simulink model "Series"  (R2020a)
settings: Solver=VariableStepAuto  StartTime=0.0  StopTime=6948  RelTol=1e-3
values from neighbouring files (symbols this model uses):
  diff_gear = 4.51    [Series_script.m]
  gear_down = []    [Series_script.m]
  gear_eff = 0.98    [Series_script.m]
  gear_idling_loss = 0    [Series_script.m]
  gear_ratio = [1]    [Series_script.m]
  gear_up = []    [Series_script.m]
  Gears = 1    [Series_script.m]
  max_battery = 0.6*150*1000    (= 90000)    [Series_script.m]
  max_CE_power = 48    [Series_script.m]
  max_EG_power = 35    [Series_script.m]
  max_EM_power = 150    [Series_script.m]
  max_SOC = 0.60    (= 0.6)    [Series_script.m]
  min_SOC = 0.30    (= 0.3)    [Series_script.m]
  Series_add_Mass = 250    [Series_script.m]
  T_CE_max = p_me_max.*V_d/(2*pi*2)    [Eng_plot.m]
  T_EG_max = max_EG_power *1000 / max_EG_power_old * T_EG_max    [Gen_plot.m]
  T_EM_max = max_EM_power *1000 / max_EM_power_old * T_EM_max    [motor_plot.m]
  V_Mass = 1920    [Series_script.m]
  V_wheel_dia = 0.739    [Series_script.m]
undefined symbols (not defined in the file or in its folder): automatic_gearbox, eta_EG_map, eta_EM_map, H_u, P_aux, P_CE_cutoff, P_CE_idle, r, T_CE_cutoff, theta_CE, theta_EM, V_CE_map, w_CE_idle, w_CE_max, w_CE_upper, w_EG_row, w_EG_upper, w_EM_row, w_EM_upper
libraries: qss_tb_library x6, simulink x1
settings Model: Creator=Rahul Pai  LastModifiedBy=Rahul Pai

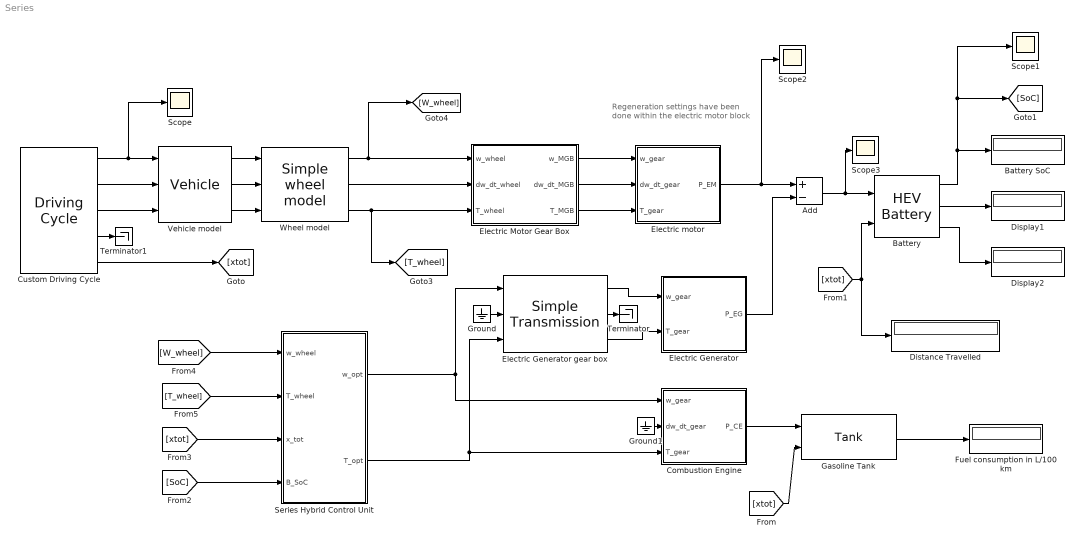
== system Series ==
  note: Regeneration settings have been
      | done within the electric motor block
  Add : Sum  Inputs=+-
  Battery : qss_tb_library/Energy Buffer/HEV Battery  Tag=battery  cell_series=N_series  cell_parallel=N_parallel  Q_BT_IC_rel=Init_SoC
  Battery SoC : Display
  Combustion Engine : Subsystem  Tag=combustion engine  AncestorBlock=qss_tb_library/Energy Converter/CE Assignment  mask(Combustion Engine (based on consumption map)){engine_type=Gasoline, P_ice=max_CE_power, ENABLE_FUEL_CUTOFF=on}
      mask prompts: engine_type "Engine type"; P_ice "Power [kW]"; ENABLE_FUEL_CUTOFF "Enable fuel cutoff"
      mask help:
      | This block simulates the behaviour of a combustion engine. The block is based on consumption maps for medium sized passenger cars.
      |
      | NA Gasoline:
      | max power @ 5000 rpm
      | max torque @ 3000 rpm
      |
      | Small Diesel:
      | max power @ 4500 rpm
      | max torque @ 2000 rpm
      |
      | Large Diesel:
      | max power @ 1500 rpm
      | max torque @ 1500 rpm
      |
      |
      | Input:
      | =====
      | 	w_gear	Speed of the fly wheel [rad/s]
      | 	dw_dt_gear	Acceleration of the fly wheel [rad/s^2]
      | 	T_gear	Torque on the fly wheel [Nm]
      |
      | Output:
      | ======
      | 	P_CE	Fuel power consumed by the combustion engine [W]
      mask init:
      | init_AssCE_map;
      mask TypeOptions engine_type: Gasoline | Small Diesel | Large Diesel
  Custom Driving Cycle : qss_tb_library/Driving Cycle/Driving Cycle  Tag=cycle  cyclename1=Assignment_2_cycle  stepsize=1  autostop=on
  Display1 : Display
  Display2 : Display
  Distance Travelled : Display
      settings: Format=decimal (Stored Integer)
  Electric Generator : Subsystem  AncestorBlock=qss_tb_library/Energy Converter/EG Assignment  mask(Electric Generator){P_eg=max_EG_power}
      mask prompts: P_eg "Maximum mechanical power [kW]"
      mask help:
      | This block simulates the behaviour of an electric generator. The block is based on an efficiency map.
      |
      | Input:
      | =====
      | 	w_gear	Speed of the generator [rad/s]
      | 	T_gear	Torque of the generator [Nm]
      |
      | Output:
      | ======
      | 	P_EG	Electric power of the generator [W]
      |
      | Generator map:
      | ======
      | The generator map file must contain the following variables:
      | eta_EG_map		% Efficiency map                    [-]
      | w_EG_row                        % Generator speed range             [rad/s]
      | T_EG_col		% Generator torque range            [Nm]
      | w_EG_max		% Maximum generator speed           [rad/s]
      | T_EG_max		% Maximum generator torque          [Nm]
      |
      | ======
      mask init:
      | init_EG_ass;
  Electric Generator gear box : qss_tb_library/Gear System/Simple Transmission  Tag=simple transmission  gear_ratio=EM_gear_ratio  e_GT=EM_gear_eta  P_GT0=EM_idling_loss  w_wheel_min=1
  Electric Motor Gear Box : Subsystem  Tag=transmission  AncestorBlock=qss_tb_library/Gear System/Automatic Gear Box  mask(Automatic Gear Box){nog=Gears, i=gear_ratio, i_diff=diff_gear, gearon=gear_up, gearoff=gear_down, d=V_wheel_dia, e_GT=gear_eff, P_GT0=gear_idling_loss, w_wheel_min=1}
      mask prompts: nog "Number of gears"; i "Gear ratio vector"; i_diff "Differential gear [-]"; gearon "Switching points for upshift [km/h]"; gearoff "Switching points for downshift [km/h]"; d "Wheel diameter"; e_GT "Efficiency [-]"; P_GT0 "Idling losses (friction) [W]"; w_wheel_min "Minimum wheel speed beyond which losses are generated [rad/s]"
      mask help:
      | This block simulates a automatic gear box, can handle up to 16 gears.
      |
      | Input:
      | =====
      | 	w_wheel	Speed of the wheel [rad/s]
      | 	dw_dt_wheel	Acceleration of the wheel [rad/s^2],
      | 	T_wheel	Torque on the wheel [Nm]
      | 	i	Gear number [-]
      |
      | Output:
      | ======
      | 	w_MGB	Speed of the fly wheel [rad/s]
      | 	dw_dt_MGB	Acceleration of the fly wheel [rad/s^2]
      | 	T_MGB	Torque on the fly wheel [Nm]
      |
      | Number of gears:
      | ======
      | Specify the number of forward gears
      |
      | Shifting points for upshift:
      | ======
      | Vector specifying the velocity for shifting
      | [first_to_second_gear    second_to_third_gear    ....]
      | The number of elements in the vector should be Number of gears - 1.
      |
      | Shifting points for udownshift:
      | ======
      | Simular to upshift
      | [second_to_first_gear    third_to_second_gear    ....]
      mask init:
      | init_AGB;
  Electric motor : Subsystem  AncestorBlock=qss_tb_library/Energy Converter/EM Assignment  mask(Electric Motor){P_em=max_EM_power}
      mask prompts: P_em "Power [kW]"
      mask help:
      | This block simulates the behaviour of an electric motor. The block is based on an efficiency map. The map is located in the Data/EnergyConvertter/ElectricMotor directory.
      |
      | Maximum speed och the electric motor is 6000 rpm
      | Field weakening region starts at 1500 rpm
      | Maximum mechanical power is at 2150 rpm
      | The maximum torque is 5.98 Nm/kW multiplied with the power you select.
      |
      | Input:
      | =====
      | 	w_gear	Speed of the motor [rad/s]
      | 	dw_dt_gear	Acceleration of the motor [rad/s^2]
      | 	T_gear	Torque of the motor [Nm]
      |
      | Output:
      | ======
      | 	P_EM	Electric Power consumed by the  motor [W]
      mask init:
      | init_EM_ass;
  Fuel consumption in L/100 km : Display
  Gasoline Tank : qss_tb_library/Energy Source/Tank  Tag=tank  fuel=Gasoline  flag_cold_start=on
  Ground : Ground
  Ground1 : Ground
  Scope{,1..3} (4 alike) : Scope
  Series Hybrid Control Unit : Subsystem  Tag=control unit  AncestorBlock=|  mask(Control Unit){}
      | qss_tb_library/Controller/Control Unit
      | (empty template)
      mask help:
      | This block gives the user the opportunity to design his/her own control unit.
      |
      | The user can define the inputs and outputs  by himself/herself.
  Terminator : Terminator
  Terminator1 : Terminator
  Vehicle model : qss_tb_library/Vehicle/Vehicle  Tag=vehicle  m_f=V_Mass+Series_add_Mass  A_f=V_area  cw=V_d  mu=V_RRC  k_inertia=V_Rotating
  Wheel model : qss_tb_library/Vehicle/Simple wheel model  Tag=simple transmission  d_wheel=V_wheel_dia
  wires:
  Custom Driving Cycle/1 -> Scope/1, Vehicle model/1
  Custom Driving Cycle/2 -> Vehicle model/2
  Custom Driving Cycle/3 -> Vehicle model/3
  Vehicle model/1 -> Wheel model/1
  Vehicle model/2 -> Wheel model/2
  Vehicle model/3 -> Wheel model/3
  Wheel model/1 -> [W_wheel], Electric Motor Gear Box/1(w_wheel)
  Wheel model/2 -> Electric Motor Gear Box/2(dw_dt_wheel)
  Electric Motor Gear Box/1(w_MGB) -> Electric motor/1(w_gear)
  Electric Motor Gear Box/2(dw_dt_MGB) -> Electric motor/2(dw_dt_gear)
  Electric Motor Gear Box/3(T_MGB) -> Electric motor/3(T_gear)
  Electric motor/1(P_EM) -> Scope2/1, Add/1
  Battery/1 -> Scope1/1, [SoC], Battery SoC/1
  Battery/2 -> Display1/1
  Battery/3 -> Display2/1
  Gasoline Tank/1 -> Fuel consumption in L/100 km/1
  Combustion Engine/1(P_CE) -> Gasoline Tank/1
  Electric Generator gear box/1 -> Electric Generator/1(w_gear)
  Electric Generator gear box/3 -> Electric Generator/2(T_gear)
  Electric Generator gear box/2 -> Terminator/1
  Ground/1 -> Electric Generator gear box/2
  Ground1/1 -> Combustion Engine/2(dw_dt_gear)
  Custom Driving Cycle/5 -> [xtot]
  [xtot] -> Gasoline Tank/2
  [xtot] -> Battery/2, Distance Travelled/1
  Electric Generator/1(P_EG) -> Add/2
  Add/1 -> Scope3/1, Battery/1
  Series Hybrid Control Unit/1(w_opt) -> Combustion Engine/1(w_gear), Electric Generator gear box/1
  Series Hybrid Control Unit/2(T_opt) -> Electric Generator gear box/3, Combustion Engine/3(T_gear)
  [SoC] -> Series Hybrid Control Unit/4(B_SoC)
  [xtot] -> Series Hybrid Control Unit/3(x_tot)
  Wheel model/3 -> [T_wheel], Electric Motor Gear Box/3(T_wheel)
  Custom Driving Cycle/4 -> Terminator1/1
  [T_wheel] -> Series Hybrid Control Unit/2(T_wheel)
  [W_wheel] -> Series Hybrid Control Unit/1(w_wheel)

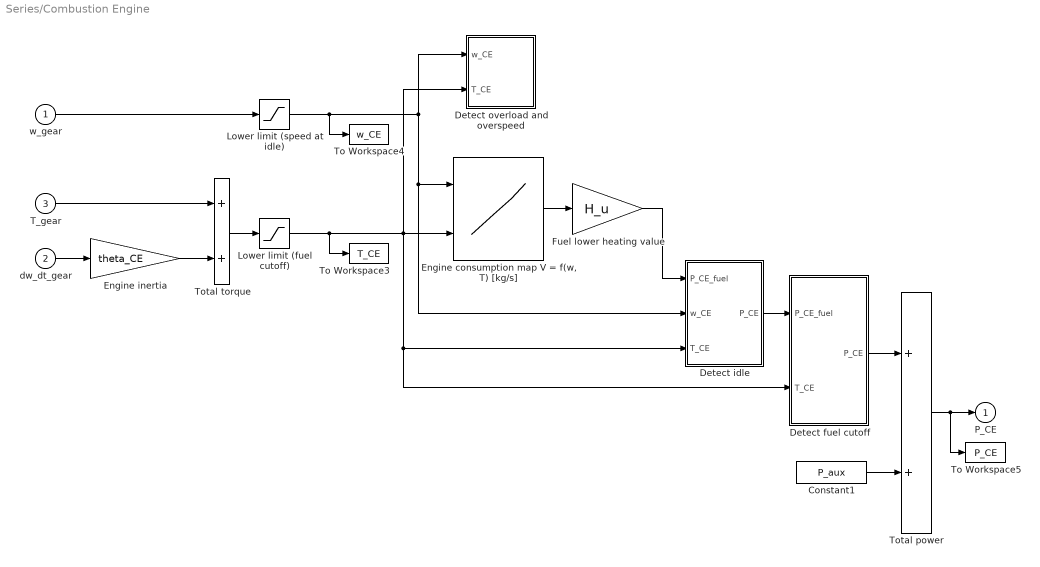
== system Series/Combustion Engine ==
  w_gear : Inport
  dw_dt_gear : Inport  Port=2
  T_gear : Inport  Port=3
  Constant1 : Constant  Value=P_aux
  Detect fuel cutoff : Subsystem
  Detect idle : Subsystem
  Detect overload and overspeed : Subsystem
  "Engine consumption map V = f(w, T) [kg/s]" : Lookup2D  RowIndex=w_CE_row  ColumnIndex=T_CE_col  Table=V_CE_map
  Engine inertia : Gain  Gain=theta_CE  SaturateOnIntegerOverflow=on  OutDataTypeStr=Inherit: Same as input  ParamDataTypeStr=Inherit: Same as input
  Fuel lower heating value : Gain  Gain=H_u  SaturateOnIntegerOverflow=on  OutDataTypeStr=Inherit: Same as input  ParamDataTypeStr=Inherit: Same as input
  Lower limit (fuel cutoff) : Saturate  UpperLimit=inf  LowerLimit=T_CE_cutoff
  Lower limit (speed at idle) : Saturate  UpperLimit=inf  LowerLimit=w_CE_idle
  To Workspace3 : ToWorkspace  VariableName=T_CE  SampleTime=-1
  To Workspace4 : ToWorkspace  VariableName=w_CE  SampleTime=-1
  To Workspace5 : ToWorkspace  VariableName=P_CE  SampleTime=-1
  Total power : Sum  InputSameDT=on  SaturateOnIntegerOverflow=on  OutDataTypeStr=Inherit: Same as first input
  Total torque : Sum  InputSameDT=on  SaturateOnIntegerOverflow=on  OutDataTypeStr=Inherit: Same as first input
  P_CE : Outport  InitialOutput=0
  wires:
  T_gear/1 -> Total torque/1
  dw_dt_gear/1 -> Engine inertia/1
  Total torque/1 -> Lower limit (fuel cutoff)/1
  Engine inertia/1 -> Total torque/2
  Lower limit (speed at idle)/1 -> Detect overload and overspeed/1(w_CE), Detect idle/2(w_CE), "Engine consumption map V = f(w, T) [kg/s]"/1, To Workspace4/1
  w_gear/1 -> Lower limit (speed at idle)/1
  Fuel lower heating value/1 -> Detect idle/1(P_CE_fuel)
  Detect idle/1(P_CE) -> Detect fuel cutoff/1(P_CE_fuel)
  "Engine consumption map V = f(w, T) [kg/s]"/1 -> Fuel lower heating value/1
  Detect fuel cutoff/1(P_CE) -> Total power/1
  Total power/1 -> P_CE/1, To Workspace5/1
  Constant1/1 -> Total power/2
  Lower limit (fuel cutoff)/1 -> Detect overload and overspeed/2(T_CE), "Engine consumption map V = f(w, T) [kg/s]"/2, Detect idle/3(T_CE), Detect fuel cutoff/2(T_CE), To Workspace3/1

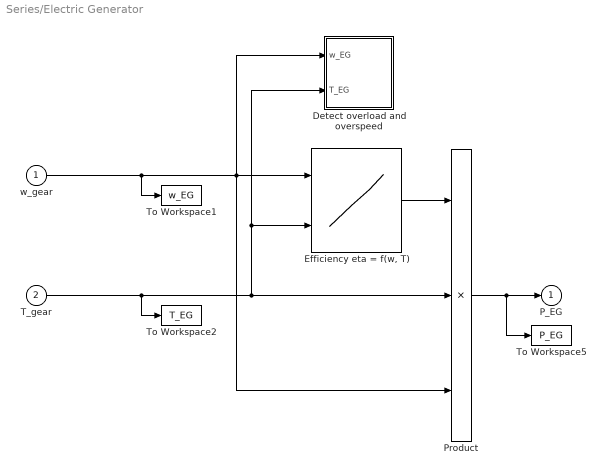
== system Series/Electric Generator ==
  w_gear : Inport
  T_gear : Inport  Port=2
  Detect overload and overspeed : Subsystem
  "Efficiency eta = f(w, T)" : Lookup2D  RowIndex=w_EG_row  ColumnIndex=T_EG_col  Table=eta_EG_map
  Product : Product  Inputs=3  InputSameDT=on  RndMeth=Zero  SaturateOnIntegerOverflow=on  OutDataTypeStr=Inherit: Same as first input
  To Workspace1 : ToWorkspace  VariableName=w_EG  SampleTime=-1
  To Workspace2 : ToWorkspace  VariableName=T_EG  SampleTime=-1
  To Workspace5 : ToWorkspace  VariableName=P_EG  SampleTime=-1
  P_EG : Outport  InitialOutput=0
  wires:
  w_gear/1 -> To Workspace1/1, Detect overload and overspeed/1(w_EG), "Efficiency eta = f(w, T)"/1, Product/3
  Product/1 -> To Workspace5/1, P_EG/1
  "Efficiency eta = f(w, T)"/1 -> Product/1
  T_gear/1 -> To Workspace2/1, Detect overload and overspeed/2(T_EG), "Efficiency eta = f(w, T)"/2, Product/2

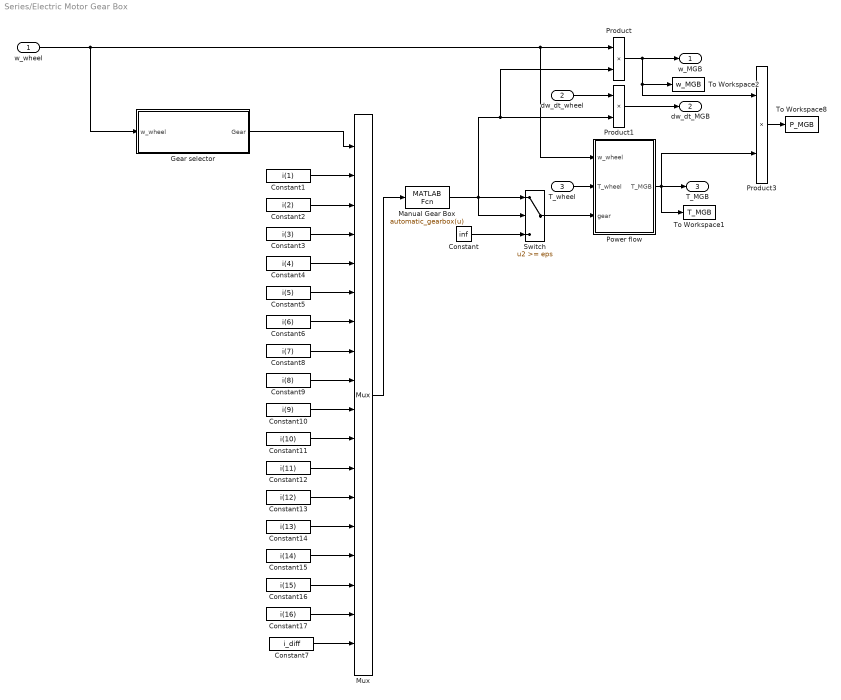
== system Series/Electric Motor Gear Box ==
  w_wheel : Inport
  dw_dt_wheel : Inport  Port=2
  T_wheel : Inport  Port=3
  Constant : Constant  Value=inf
  Constant1 : Constant  Value=i(1)
  Constant10 : Constant  Value=i(9)
  Constant11 : Constant  Value=i(10)
  Constant12 : Constant  Value=i(11)
  Constant13 : Constant  Value=i(12)
  Constant14 : Constant  Value=i(13)
  Constant15 : Constant  Value=i(14)
  Constant16 : Constant  Value=i(15)
  Constant17 : Constant  Value=i(16)
  Constant2 : Constant  Value=i(2)
  Constant3 : Constant  Value=i(3)
  Constant4 : Constant  Value=i(4)
  Constant5 : Constant  Value=i(5)
  Constant6 : Constant  Value=i(6)
  Constant7 : Constant  Value=i_diff
  Constant8 : Constant  Value=i(7)
  Constant9 : Constant  Value=i(8)
  Gear selector : Subsystem
  Manual Gear Box : MATLABFcn  MATLABFcn=automatic_gearbox(u)  OutputDimensions=1
  Mux : Mux  Inputs=18
  Power flow : Subsystem
  Product : Product  InputSameDT=on  RndMeth=Zero  SaturateOnIntegerOverflow=on  OutDataTypeStr=Inherit: Same as first input
  Product1 : Product  InputSameDT=on  RndMeth=Zero  SaturateOnIntegerOverflow=on  OutDataTypeStr=Inherit: Same as first input
  Product3 : Product  InputSameDT=on  RndMeth=Zero  SaturateOnIntegerOverflow=on  OutDataTypeStr=Inherit: Same as first input
  Switch : Switch  Threshold=eps  SaturateOnIntegerOverflow=on  InputSameDT=on
  To Workspace1 : ToWorkspace  VariableName=T_MGB  SampleTime=-1
  To Workspace2 : ToWorkspace  VariableName=w_MGB  SampleTime=-1
  To Workspace8 : ToWorkspace  VariableName=P_MGB  SampleTime=-1
  w_MGB : Outport  InitialOutput=0
  dw_dt_MGB : Outport  Port=2  InitialOutput=0
  T_MGB : Outport  Port=3  InitialOutput=0
  wires:
  Constant17/1 -> Mux/17
  Constant16/1 -> Mux/16
  Constant15/1 -> Mux/15
  Constant14/1 -> Mux/14
  Constant13/1 -> Mux/13
  Constant12/1 -> Mux/12
  Constant11/1 -> Mux/11
  Constant10/1 -> Mux/10
  Constant9/1 -> Mux/9
  Constant8/1 -> Mux/8
  Constant7/1 -> Mux/18
  Power flow/1(T_MGB) -> T_MGB/1, Product3/2, To Workspace1/1
  Product/1 -> w_MGB/1, Product3/1, To Workspace2/1
  Constant/1 -> Switch/3
  w_wheel/1 -> Gear selector/1(w_wheel), Product/1, Power flow/1(w_wheel)
  Product1/1 -> dw_dt_MGB/1
  dw_dt_wheel/1 -> Product1/1
  Manual Gear Box/1 -> Product/2, Product1/2, Switch/2, Switch/1
  Product3/1 -> To Workspace8/1
  Switch/1 -> Power flow/3(gear)
  T_wheel/1 -> Power flow/2(T_wheel)
  Constant1/1 -> Mux/2
  Constant2/1 -> Mux/3
  Constant3/1 -> Mux/4
  Constant4/1 -> Mux/5
  Constant5/1 -> Mux/6
  Constant6/1 -> Mux/7
  Gear selector/1(Gear) -> Mux/1
  Mux/1 -> Manual Gear Box/1

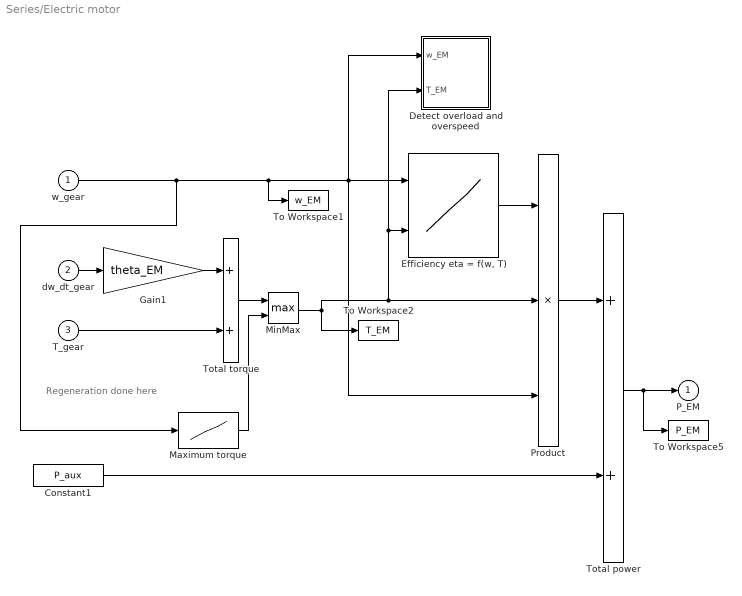
== system Series/Electric motor ==
  note: Regeneration done here
  w_gear : Inport
  dw_dt_gear : Inport  Port=2
  T_gear : Inport  Port=3
  Constant1 : Constant  Value=P_aux
  Detect overload and overspeed : Subsystem
  "Efficiency eta = f(w, T)" : Lookup2D  RowIndex=w_EM_row  ColumnIndex=T_EM_col  Table=eta_EM_map
  Gain1 : Gain  Gain=theta_EM  SaturateOnIntegerOverflow=on  OutDataTypeStr=Inherit: Same as input  ParamDataTypeStr=Inherit: Same as input
  Maximum torque : Lookup  InputValues=w_EM_row  Table=-T_EM_max  SaturateOnIntegerOverflow=on
  MinMax : MinMax  Function=max  Inputs=2
  Product : Product  Inputs=3  InputSameDT=on  RndMeth=Zero  SaturateOnIntegerOverflow=on  OutDataTypeStr=Inherit: Same as first input
  To Workspace1 : ToWorkspace  VariableName=w_EM  SampleTime=-1
  To Workspace2 : ToWorkspace  VariableName=T_EM  SampleTime=-1
  To Workspace5 : ToWorkspace  VariableName=P_EM  SampleTime=-1
  Total power : Sum  InputSameDT=on  SaturateOnIntegerOverflow=on  OutDataTypeStr=Inherit: Same as first input
  Total torque : Sum  InputSameDT=on  SaturateOnIntegerOverflow=on  OutDataTypeStr=Inherit: Same as first input
  P_EM : Outport  InitialOutput=0
  wires:
  Total power/1 -> To Workspace5/1, P_EM/1
  Product/1 -> Total power/1
  Constant1/1 -> Total power/2
  MinMax/1 -> To Workspace2/1, Product/2, "Efficiency eta = f(w, T)"/2, Detect overload and overspeed/2(T_EM)
  Gain1/1 -> Total torque/1
  T_gear/1 -> Total torque/2
  dw_dt_gear/1 -> Gain1/1
  "Efficiency eta = f(w, T)"/1 -> Product/1
  w_gear/1 -> Maximum torque/1, To Workspace1/1, Product/3, "Efficiency eta = f(w, T)"/1, Detect overload and overspeed/1(w_EM)
  Total torque/1 -> MinMax/1
  Maximum torque/1 -> MinMax/2

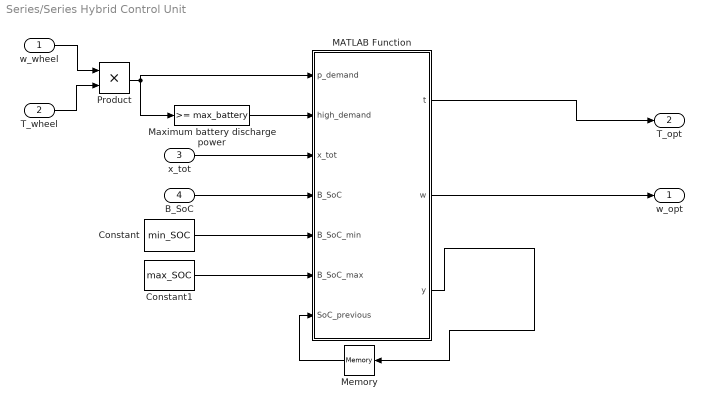
== system Series/Series Hybrid Control Unit ==
  w_wheel : Inport
  T_wheel : Inport  Port=2
  x_tot : Inport  Port=3
  B_SoC : Inport  Port=4
  Constant : Constant  Value=min_SOC
  Constant1 : Constant  Value=max_SOC
  MATLAB Function : MATLAB Function  TreatAsAtomicUnit=on
  Maximum battery discharge power : simulink/Logic and Bit Operations/Compare To Constant  relop=>=  const=max_battery  OutDataTypeStr=boolean
  Memory : Memory
  Product : Product
  w_opt : Outport  InitialOutput=0
  T_opt : Outport  Port=2  InitialOutput=0
  wires:
  Memory/1 -> MATLAB Function/7(SoC_previous)
  x_tot/1 -> MATLAB Function/3(x_tot)
  Constant/1 -> MATLAB Function/5(B_SoC_min)
  B_SoC/1 -> MATLAB Function/4(B_SoC)
  MATLAB Function/3(y) -> Memory/1
  Constant1/1 -> MATLAB Function/6(B_SoC_max)
  MATLAB Function/2(w) -> w_opt/1
  MATLAB Function/1(t) -> T_opt/1
  w_wheel/1 -> Product/1
  T_wheel/1 -> Product/2
  Product/1 -> Maximum battery discharge power/1, MATLAB Function/1(p_demand)
  Maximum battery discharge power/1 -> MATLAB Function/2(high_demand)

== system Series/Combustion Engine/Detect fuel cutoff ==
  P_CE_fuel : Inport
  T_CE : Inport  Port=2
  Constant1 : Constant  Value=ENABLE_FUEL_CUTOFF
  Constant3 : Constant  Value=P_CE_cutoff
  Decision : Switch  Threshold=0.5
  Detect fuel cutoff : Switch  Threshold=T_CE_cutoff + 0.01  SaturateOnIntegerOverflow=on  InputSameDT=on
  P_CE : Outport
  wires:
  Constant3/1 -> Detect fuel cutoff/3
  T_CE/1 -> Detect fuel cutoff/2
  P_CE_fuel/1 -> Detect fuel cutoff/1, Decision/3
  Detect fuel cutoff/1 -> Decision/1
  Constant1/1 -> Decision/2
  Decision/1 -> P_CE/1

== system Series/Combustion Engine/Detect idle ==
  P_CE_fuel : Inport
  w_CE : Inport  Port=2
  T_CE : Inport  Port=3
  Constant3 : Constant  Value=P_CE_idle
  Idle detection : Fcn  Expr=(u(1) <= w_CE_idle) * (u(2) <= T_CE_idle)
  Mux : Mux  Inputs=2
  Switch2 : Switch  Threshold=0.5  SaturateOnIntegerOverflow=on  InputSameDT=on
  P_CE : Outport  InitialOutput=0
  wires:
  Mux/1 -> Idle detection/1
  T_CE/1 -> Mux/2
  w_CE/1 -> Mux/1
  Idle detection/1 -> Switch2/2
  P_CE_fuel/1 -> Switch2/3
  Switch2/1 -> P_CE/1
  Constant3/1 -> Switch2/1

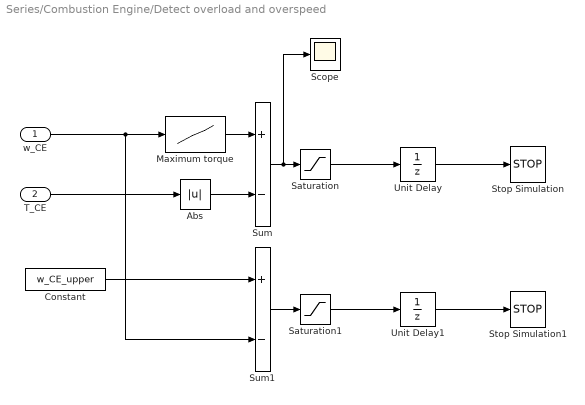
== system Series/Combustion Engine/Detect overload and overspeed ==
  w_CE : Inport
  T_CE : Inport  Port=2
  Abs : Abs  SaturateOnIntegerOverflow=on
  Constant : Constant  Value=w_CE_upper
  Maximum torque : Lookup  InputValues=w_CE_max  Table=T_CE_max  SaturateOnIntegerOverflow=on
  Saturation : Saturate  UpperLimit=0  LowerLimit=-inf
  Saturation1 : Saturate  UpperLimit=0  LowerLimit=-inf
  Scope : Scope
  Stop Simulation : Stop
  Stop Simulation1 : Stop
  Sum : Sum  Inputs=+-  InputSameDT=on  SaturateOnIntegerOverflow=on  OutDataTypeStr=Inherit: Same as first input
  Sum1 : Sum  Inputs=+-  InputSameDT=on  SaturateOnIntegerOverflow=on  OutDataTypeStr=Inherit: Same as first input
  Unit Delay : UnitDelay  SampleTime=-1  HasFrameUpgradeWarning=on
  Unit Delay1 : UnitDelay  SampleTime=-1  HasFrameUpgradeWarning=on
  wires:
  Sum/1 -> Scope/1, Saturation/1
  w_CE/1 -> Maximum torque/1, Sum1/2
  T_CE/1 -> Abs/1
  Maximum torque/1 -> Sum/1
  Abs/1 -> Sum/2
  Saturation/1 -> Unit Delay/1
  Constant/1 -> Sum1/1
  Sum1/1 -> Saturation1/1
  Saturation1/1 -> Unit Delay1/1
  Unit Delay/1 -> Stop Simulation/1
  Unit Delay1/1 -> Stop Simulation1/1

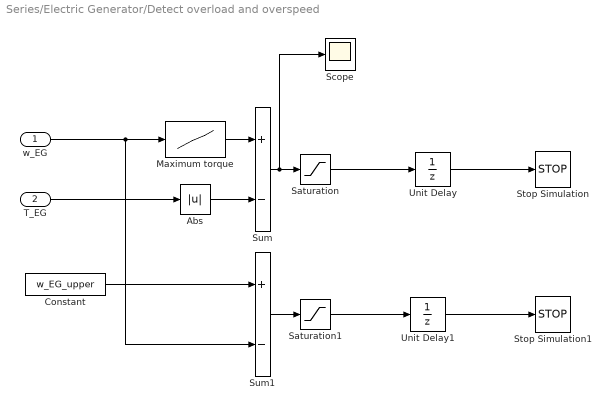
== system Series/Electric Generator/Detect overload and overspeed ==
  w_EG : Inport
  T_EG : Inport  Port=2
  Abs : Abs  SaturateOnIntegerOverflow=on
  Constant : Constant  Value=w_EG_upper
  Maximum torque : Lookup  InputValues=w_EG_row  Table=T_EG_max  SaturateOnIntegerOverflow=on
  Saturation : Saturate  UpperLimit=0  LowerLimit=-inf
  Saturation1 : Saturate  UpperLimit=0  LowerLimit=-inf
  Scope : Scope
  Stop Simulation : Stop
  Stop Simulation1 : Stop
  Sum : Sum  Inputs=+-  InputSameDT=on  SaturateOnIntegerOverflow=on  OutDataTypeStr=Inherit: Same as first input
  Sum1 : Sum  Inputs=+-  InputSameDT=on  SaturateOnIntegerOverflow=on  OutDataTypeStr=Inherit: Same as first input
  Unit Delay : UnitDelay  SampleTime=-1  HasFrameUpgradeWarning=on
  Unit Delay1 : UnitDelay  SampleTime=-1  HasFrameUpgradeWarning=on
  wires:
  Saturation1/1 -> Unit Delay1/1
  Sum1/1 -> Saturation1/1
  Constant/1 -> Sum1/1
  Saturation/1 -> Unit Delay/1
  Abs/1 -> Sum/2
  Maximum torque/1 -> Sum/1
  T_EG/1 -> Abs/1
  w_EG/1 -> Sum1/2, Maximum torque/1
  Sum/1 -> Scope/1, Saturation/1
  Unit Delay/1 -> Stop Simulation/1
  Unit Delay1/1 -> Stop Simulation1/1

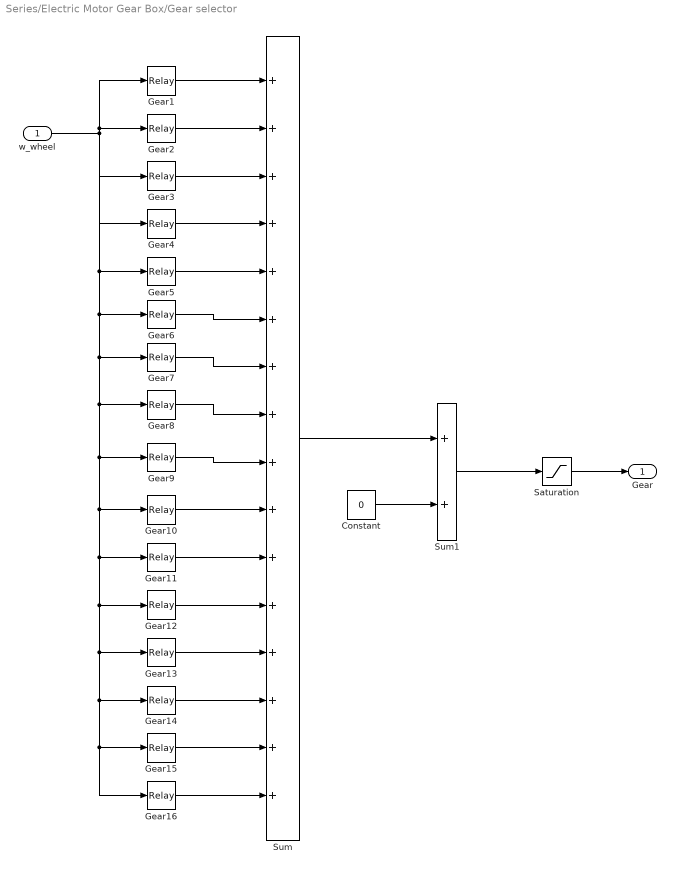
== system Series/Electric Motor Gear Box/Gear selector ==
  w_wheel : Inport
  Constant : Constant  Value=0
  Gear1 : Relay  OffSwitchValue=0
  Gear10 : Relay  OnSwitchValue=gearon(9)/3.6/r  OffSwitchValue=gearoff(9)/3.6/r
  Gear11 : Relay  OnSwitchValue=gearon(10)/3.6/r  OffSwitchValue=gearoff(10)/3.6/r
  Gear12 : Relay  OnSwitchValue=gearon(11)/3.6/r  OffSwitchValue=gearoff(11)/3.6/r
  Gear13 : Relay  OnSwitchValue=gearon(12)/3.6/r  OffSwitchValue=gearoff(12)/3.6/r
  Gear14 : Relay  OnSwitchValue=gearon(13)/3.6/r  OffSwitchValue=gearoff(13)/3.6/r
  Gear15 : Relay  OnSwitchValue=gearon(14)/3.6/r  OffSwitchValue=gearoff(14)/3.6/r
  Gear16 : Relay  OnSwitchValue=gearon(15)/3.6/r  OffSwitchValue=gearoff(15)/3.6/r
  Gear2 : Relay  OnSwitchValue=gearon(1)/3.6/r  OffSwitchValue=gearoff(1)/3.6/r
  Gear3 : Relay  OnSwitchValue=gearon(2)/3.6/r  OffSwitchValue=gearoff(2)/3.6/r
  Gear4 : Relay  OnSwitchValue=gearon(3)/3.6/r  OffSwitchValue=gearoff(3)/3.6/r
  Gear5 : Relay  OnSwitchValue=gearon(4)/3.6/r  OffSwitchValue=gearoff(4)/3.6/r
  Gear6 : Relay  OnSwitchValue=gearon(5)/3.6/r  OffSwitchValue=gearoff(5)/3.6/r
  Gear7 : Relay  OnSwitchValue=gearon(6)/3.6/r  OffSwitchValue=gearoff(6)/3.6/r
  Gear8 : Relay  OnSwitchValue=gearon(7)/3.6/r  OffSwitchValue=gearoff(7)/3.6/r
  Gear9 : Relay  OnSwitchValue=gearon(8)/3.6/r  OffSwitchValue=gearoff(8)/3.6/r
  Saturation : Saturate  UpperLimit=nog  LowerLimit=0
  Sum : Sum  Inputs=16  SaturateOnIntegerOverflow=on
  Sum1 : Sum  Inputs=2  SaturateOnIntegerOverflow=on
  Gear : Outport
  wires:
  Saturation/1 -> Gear/1
  Gear6/1 -> Sum/6
  Gear7/1 -> Sum/7
  Gear8/1 -> Sum/8
  Gear9/1 -> Sum/9
  Gear10/1 -> Sum/10
  Gear11/1 -> Sum/11
  Gear12/1 -> Sum/12
  Gear13/1 -> Sum/13
  Gear14/1 -> Sum/14
  Gear15/1 -> Sum/15
  Gear16/1 -> Sum/16
  Gear5/1 -> Sum/5
  w_wheel/1 -> Gear16/1, Gear15/1, Gear14/1, Gear13/1, Gear12/1, Gear11/1, Gear10/1, Gear9/1, Gear8/1, Gear7/1, Gear6/1, Gear5/1, Gear1/1, Gear2/1, Gear3/1, Gear4/1
  Gear1/1 -> Sum/1
  Gear2/1 -> Sum/2
  Gear3/1 -> Sum/3
  Gear4/1 -> Sum/4
  Sum/1 -> Sum1/1
  Sum1/1 -> Saturation/1
  Constant/1 -> Sum1/2

== system Series/Electric Motor Gear Box/Power flow ==
  w_wheel : Inport
  T_wheel : Inport  Port=2
  gear : Inport  Port=3
  "Engine -> Wheel" : Subsystem
  Switch1 : Switch  SaturateOnIntegerOverflow=on  InputSameDT=on
  "Wheel -> Engine" : Subsystem
  T_MGB : Outport  InitialOutput=0
  wires:
  w_wheel/1 -> "Wheel -> Engine"/1(w_wheel), "Engine -> Wheel"/1(w_wheel)
  gear/1 -> "Wheel -> Engine"/3(gear), "Engine -> Wheel"/3(gear)
  "Wheel -> Engine"/1(T_MGB-) -> Switch1/3
  T_wheel/1 -> "Wheel -> Engine"/2(T_wheel), "Engine -> Wheel"/2(T_wheel), Switch1/2
  "Engine -> Wheel"/1(T_MGB+) -> Switch1/1
  Switch1/1 -> T_MGB/1

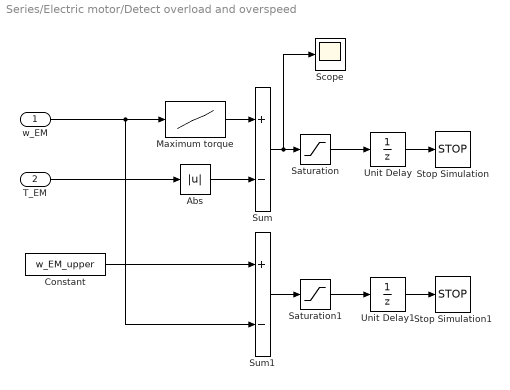
== system Series/Electric motor/Detect overload and overspeed ==
  w_EM : Inport
  T_EM : Inport  Port=2
  Abs : Abs  SaturateOnIntegerOverflow=on
  Constant : Constant  Value=w_EM_upper
  Maximum torque : Lookup  InputValues=w_EM_row  Table=T_EM_max  SaturateOnIntegerOverflow=on
  Saturation : Saturate  UpperLimit=0  LowerLimit=-inf
  Saturation1 : Saturate  UpperLimit=0  LowerLimit=-inf
  Scope : Scope
  Stop Simulation : Stop
  Stop Simulation1 : Stop
  Sum : Sum  Inputs=+-  InputSameDT=on  SaturateOnIntegerOverflow=on  OutDataTypeStr=Inherit: Same as first input
  Sum1 : Sum  Inputs=+-  InputSameDT=on  SaturateOnIntegerOverflow=on  OutDataTypeStr=Inherit: Same as first input
  Unit Delay : UnitDelay  SampleTime=-1  HasFrameUpgradeWarning=on
  Unit Delay1 : UnitDelay  SampleTime=-1  HasFrameUpgradeWarning=on
  wires:
  Sum/1 -> Scope/1, Saturation/1
  w_EM/1 -> Maximum torque/1, Sum1/2
  T_EM/1 -> Abs/1
  Maximum torque/1 -> Sum/1
  Abs/1 -> Sum/2
  Saturation/1 -> Unit Delay/1
  Constant/1 -> Sum1/1
  Sum1/1 -> Saturation1/1
  Saturation1/1 -> Unit Delay1/1
  Unit Delay/1 -> Stop Simulation/1
  Unit Delay1/1 -> Stop Simulation1/1

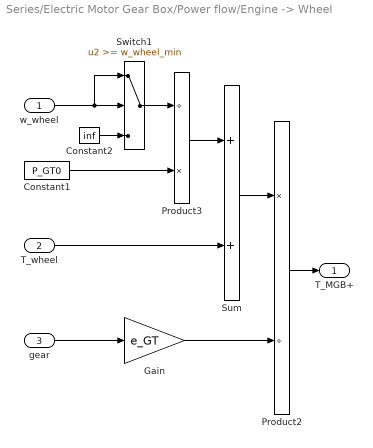
== system Series/Electric Motor Gear Box/Power flow/Engine -> Wheel ==
  w_wheel : Inport
  T_wheel : Inport  Port=2
  gear : Inport  Port=3
  Constant1 : Constant  Value=P_GT0
  Constant2 : Constant  Value=inf
  Gain : Gain  Gain=e_GT  SaturateOnIntegerOverflow=on  OutDataTypeStr=Inherit: Same as input  ParamDataTypeStr=Inherit: Same as input
  Product2 : Product  Inputs=*/  InputSameDT=on  RndMeth=Zero  SaturateOnIntegerOverflow=on  OutDataTypeStr=Inherit: Same as first input
  Product3 : Product  Inputs=/*  InputSameDT=on  RndMeth=Zero  SaturateOnIntegerOverflow=on  OutDataTypeStr=Inherit: Same as first input
  Sum : Sum  InputSameDT=on  SaturateOnIntegerOverflow=on  OutDataTypeStr=Inherit: Same as first input
  Switch1 : Switch  Threshold=w_wheel_min  SaturateOnIntegerOverflow=on  InputSameDT=on
  T_MGB+ : Outport  InitialOutput=0
  wires:
  T_wheel/1 -> Sum/2
  Product3/1 -> Sum/1
  Gain/1 -> Product2/2
  Product2/1 -> T_MGB+/1
  Sum/1 -> Product2/1
  w_wheel/1 -> Switch1/2, Switch1/1
  Constant2/1 -> Switch1/3
  Switch1/1 -> Product3/1
  Constant1/1 -> Product3/2
  gear/1 -> Gain/1

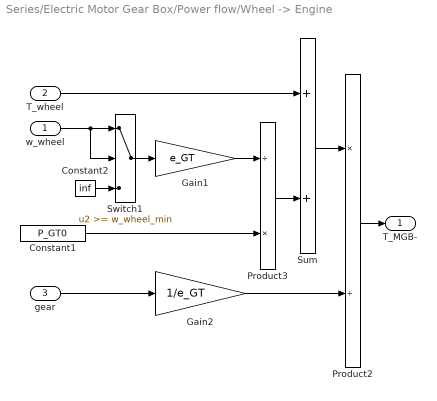
== system Series/Electric Motor Gear Box/Power flow/Wheel -> Engine ==
  w_wheel : Inport
  T_wheel : Inport  Port=2
  gear : Inport  Port=3
  Constant1 : Constant  Value=P_GT0
  Constant2 : Constant  Value=inf
  Gain1 : Gain  Gain=e_GT  SaturateOnIntegerOverflow=on  OutDataTypeStr=Inherit: Same as input  ParamDataTypeStr=Inherit: Same as input
  Gain2 : Gain  Gain=1/e_GT  SaturateOnIntegerOverflow=on  OutDataTypeStr=Inherit: Same as input  ParamDataTypeStr=Inherit: Same as input
  Product2 : Product  Inputs=*/  InputSameDT=on  RndMeth=Zero  SaturateOnIntegerOverflow=on  OutDataTypeStr=Inherit: Same as first input
  Product3 : Product  Inputs=/*  InputSameDT=on  RndMeth=Zero  SaturateOnIntegerOverflow=on  OutDataTypeStr=Inherit: Same as first input
  Sum : Sum  InputSameDT=on  SaturateOnIntegerOverflow=on  OutDataTypeStr=Inherit: Same as first input
  Switch1 : Switch  Threshold=w_wheel_min  SaturateOnIntegerOverflow=on  InputSameDT=on
  T_MGB- : Outport  InitialOutput=0
  wires:
  w_wheel/1 -> Switch1/1, Switch1/2
  gear/1 -> Gain2/1
  Constant2/1 -> Switch1/3
  Switch1/1 -> Gain1/1
  Constant1/1 -> Product3/2
  T_wheel/1 -> Sum/1
  Gain2/1 -> Product2/2
  Product2/1 -> T_MGB-/1
  Product3/1 -> Sum/2
  Sum/1 -> Product2/1
  Gain1/1 -> Product3/1

== matlab function Series/Series Hybrid Control Unit/MATLAB Function ==
  data: p_demand input; high_demand input; t output; w output; x_tot input; y output; B_SoC input; B_SoC_min input; B_SoC_max input; SoC_previous input
function [t,w,y] = fcn(p_demand,high_demand,x_tot,B_SoC,B_SoC_min,B_SoC_max,SoC_previous)
%Initiating the parameters to zero
if x_tot==1
    SoC=0;
    t=0;
    w=0;
% The controller starts from here
else
    % If the SoC of the battery is higher than the maximum SoC limit
    if B_SoC>B_SoC_max
        SoC=0;
        % The EGU is turned off
        t=0;
        w=0;
    else
        % If the SoC of the battery is lower than or even equal to the lower limit of SoC set
        if B_SoC<=B_SoC_min
            SoC=1;              % EGU is ON
            t=75.4;             % Torque request from controller
            w=2500*2*pi/60;     % The angular speed at which the torque is to be produced
            % But if the motor is regenerating
            if p_demand<=0
                %EGU is turned off
                t=0;
                w=0;
            % If the demand is above 60% of what the battery can supply
            elseif high_demand==1
                % EGU is run at a higher torque and angular speed
                t=95.25;
                w=3000*2*pi/60;
            end
        % If the SoC is in between the max and min limits set
        else
            SoC=SoC_previous;       % To check if the engine is has been running or not
            t=75.4*SoC;             % Depending on SoC previous we either provide a torque or not
            w=2500*2*pi*SoC/60;     % Depending on SoC previous we either provide an angular speed or not
            % If the motor is regenerating
            if p_demand<=0
                %EGU is turned off
                t=0;
                w=0;
            % If the demand is above 60% of what the battery can supply
            elseif high_demand==1
                % EGU is run at a higher torque and angular speed
                t=95.25;
                w=3000*2*pi/60;
            end
        end
    end
end
y = SoC;
